simulink model "ModeloSIR"  (R2020a)
settings: Solver=VariableStepAuto  StartTime=0.0  StopTime=10.0  RelTol=1e-3
values from neighbouring files (symbols this model uses):
  beta = X(1)    [ErroQuadratico.m]    (also in ErroQuadraticoSIR.m)
  I0 = 2    [ErroQuadratico.m]    (also in ErroQuadraticoSIR.m)
  r = X(2)    [ErroQuadratico.m]    (also in ErroQuadraticoSIR.m)
  R0 = 0    [ErroQuadratico.m]    (also in ErroQuadraticoSIR.m)
  S0 = 60e6    (= 60000000)    [ErroQuadratico.m]    (also in ErroQuadraticoSIR.m)
settings Model: Creator=a1  LastModifiedBy=a1

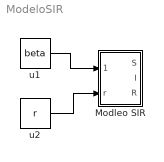
== system ModeloSIR ==
  Modleo SIR : Subsystem
  u1 : Constant  Value=beta
  u2 : Constant  Value=r
  wires:
  u1/1 -> Modleo SIR/1(beta)
  u2/1 -> Modleo SIR/2(r)

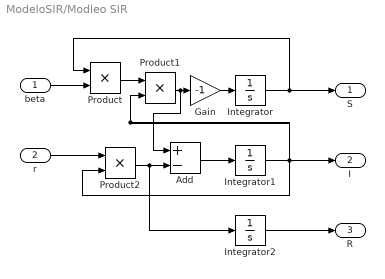
== system ModeloSIR/Modleo SIR ==
  beta : Inport
  r : Inport  Port=2
  Add : Sum  Inputs=+-
  Gain : Gain  Gain=-1
  Integrator : Integrator  InitialCondition=S0
  Integrator1 : Integrator  InitialCondition=I0
  Integrator2 : Integrator  InitialCondition=R0
  Product : Product
  Product1 : Product
  Product2 : Product
  S : Outport
  I : Outport  Port=2
  R : Outport  Port=3
  wires:
  Add/1 -> Integrator1/1
  Product2/1 -> Integrator2/1, Add/2
  r/1 -> Product2/1
  Integrator2/1 -> R/1
  Integrator/1 -> S/1, Product/1
  Product/1 -> Product1/1
  Product1/1 -> Add/1, Gain/1
  Integrator1/1 -> I/1, Product1/2, Product2/2
  Gain/1 -> Integrator/1
  beta/1 -> Product/2
